simulink model "AirRefueling_Platform_PBVS_origin"  (R2022b)
settings: Solver=ode4  StartTime=0.0  StopTime=70  FixedStep=0.02  RelTol=1e-5  AbsTol=1e-4  EnableMultiTasking=on
InitFcn:
  | F16_Init
values from neighbouring files (symbols this model uses):
  airSpeed = 393.720000000000    (= 393.72)    [F16_Init.m]    (also in Initialization.m)
  alpha0 = trimAlpha*180/pi    (= 6.62393794015)    [F16_Init.m]    (also in Initialization.m)
  altitude = 9843    [F16_Init.m]    (also in Initialization.m)
  b_ref = 30.0    (= 30)    [F16_Init.m]    (also in Initialization.m)
  C = [ 1,0,0,zeros(1,15) ... (first row only)    [F16_Init.m]    (also in Initialization.m = [1,0,0,zeros(1,15))
  C2m = [C(1,:) ... (first row only)    [F16_Init.m]    (also in Initialization.m)
  d_f_rc = [3.75;0;-0.86]    [F16_Init.m]
  d_pr_rc = [6.06;0.54;-0.86]    [F16_Init.m]
  DeltaP = [0,0,DeltaP_z(j)]    [PBVS_main.m]
  dLEF = 0    [F16_Init.m]    (also in Initialization.m)
  fi_flag = 1    [F16_Init.m]    (also in Initialization.m)
  Kc = [ ... (first row only)    [F16_Init.m]    (also in Initialization.m)
  Ki = zeros(4,3)    [F16_Init.m]    (also in Initialization.m)
  Kp = zeros(4,18)    [F16_Init.m]    (also in Initialization.m)
  mass = 636.94    [F16_Init.m]    (also in Initialization.m)
  p0_rc = [-14.35-6.06-6;-0.54-(2);5.12+0.86-(-2)]    [F16_Init.m]
  q = zeros(N,1)    [hose3D_n_air_Fv_correction.m]
  trim_ail = 0.00874607850103852    (= 0.00874607850104)    [F16_Init.m]    (also in Initialization.m)
  trim_control = [trim_thrust;trim_ele;trim_ail;trim_rud]    [F16_Init.m]    (also in Initialization.m)
  trim_ele = -2.97973164860638    (= -2.97973164861)    [F16_Init.m]    (also in Initialization.m)
  trim_rud = 0.0680302158182712    (= 0.0680302158183)    [F16_Init.m]    (also in Initialization.m)
  trim_state1 = [trim_state;0;0;0;0;0;0]    [F16_Init.m]    (also in Initialization.m)
  trim_thrust = 2279.08519954656    (= 2279.08519955)    [F16_Init.m]    (also in Initialization.m)
undefined symbols (not defined in the file or in its folder): F, gray, MIL, vt0
libraries: aerolibconvert2 x6, aerolibasang x4, aerolibwind2 x2, aerolibobsolete x2, visionmorphops x2, vrlib x1, simulink x1, aerolibatmos2 x1, aerolibadyn x1, aerolibanimutils x1
(part 2 of 2)

== matlab function AirRefueling_Platform_PBVS_origin/SimToVR ==
  data: t input; y output; PosPr1 input; PosTb1 input
function y = SimToVR(t,PosPr1,PosTb1)
%#codegen

%%函数名：SimToVR
%%用途  ：将软管锥套坐标输出转换为VR输入
%%输入  ：PosPr - 受油机椎管坐标， PlsTb - 软管坐标数据
%%输出  ：VrPos - 软管和受油机VR位置，VrAngle - 旋转角度输出
%%作者  ：戴训华
%%时间  ：2014/3/19

PosPr = PosPr1(1:3);
AttitudeRecei = [PosPr1(4);-PosPr1(6);PosPr1(5)-0.115609];

PosTb = PosTb1(1:60);

VrAngle = zeros(22*4,1);
VrPos = zeros(22*3,1);


for j = 1:21                        %前20为软管坐标数据，后1为软管平滑过渡处理
    if j == 1
        pX = [0, 0, 0]';            %软管起点
        pY = PosTb(3*j-2:3*j);      %软杆终点
    elseif j == 21                  %多加一段杆，做过渡
        pX = PosTb(3*j-5:3*j-3);
        pY = [PosTb(3*j-5)-0.7163*cos(8/180*pi),PosTb(3*j-4),PosTb(3*j-3)+0.7163*sin(8/180*pi)]';
    else
        pX = PosTb(3*j-5:3*j-3);
        pY = PosTb(3*j-2:3*j); 
    end
    
    pZ = (pX + pY)/2;               %中点坐标
    pZ = pZ * 8/3;                  %到VR中比例的缩放

    vAxis = [0,0,-1]';               %水平轴
    vTb = pY - pX;                  %杆的方向
    
    axis1 = null([vAxis';vTb']);%获取垂直向量
    vRot = axis1(:,1)';             %得到旋转轴
    
    if vRot(2) < 0
        vRot = -vRot;
    end
    
    VrAngle(4*j-3:4*j-1) = [vRot(1),vRot(3),vRot(2)]';
    VrAngle(4*j) = acos(vAxis'*vTb / sqrt(vAxis'*vAxis * vTb'*vTb));
    
    VrPos(3*j-2:3*j) = [pZ(1),-pZ(3),pZ(2)]';
end
%y = u;
VrAngle(85:88)=[AttitudeRecei(1);AttitudeRecei(2);AttitudeRecei(3);norm(AttitudeRecei)];
pZ = PosPr+[0.35 -0.1 -0.05]';
pZ = pZ * 8/3;
VrPos(3*22-2:3*22) = [pZ(1),-pZ(3),pZ(2)]';

VrPos(3*21-2) = VrPos(3*21-2)+0.8;
VrPos(3*21-1) = VrPos(3*21-1)+0.1;

if t<10
    if t>1
        VrPos(1:21*3) = VrPos(1:21*3)*(t-1)/9;
    else
        VrPos(1:21*3) = VrPos(1:21*3)*0;
    end
end

y = [VrAngle;VrPos];

== matlab function AirRefueling_Platform_PBVS_origin/Hose-Drogue System/Bow Wave Effect/Bow Wave Effect Function ==
  data: x input; Fx output; y input; z input; Fy output; Fz output
function [Fx,Fy,Fz] = F_rc2dr(x,y,z)

Cx1 = 91.6170;
Cx2 = 0.3220;
Cx3 = 3.8870;
Cx4 = 2.7359;
Cx5 = 2.4939;
Cx6 = 309.7709;
Cx7 = 0.3237;
Cx8 = 0.3851;
Cx9 = 1.1471;

Cy1 = 223.3210;
Cy2 = 0.2082;
Cy3 = 0.8102;
Cy4 = 0.6555;

Cz1 = 173.2021;
Cz2 = 0.2141;
Cz3 = 0.5697;
Cz4 = 0.7038;

if x > 5.6493
    Fx = 0;
elseif x > 3.0893
    Fx = Cx1*(1-Cx2*(x-Cx3)^2)*exp(-y^2/Cx4)*exp(z/Cx5);
else
    Fx = Cx1*(1-Cx2*(x-Cx3)^2)*exp(-y^2/Cx4)*exp(z/Cx5)...
       + Cx6*(1-Cx7*x)*exp(-y^2/Cx8)*exp(z/Cx9);
end

if x > 4.8031
    Fy = 0;
else
    Fy = Cy1*(1-Cy2*x)*(y*exp(-y^2/Cy3))*exp(z/Cy4);
end

if x > 4.6275
    Fz = 0;
else
    Fz = -Cz1*(1-Cz2*x)*exp(-y^2/Cz3)*exp(z/Cz4);
end

== matlab function AirRefueling_Platform_PBVS_origin/Hose-Drogue System/Total Turbulence   ==
  data: u1 input; u input; y output
function y = Dr_wnd2Frc(u1,u)
%#codegen

Ve=120;
rho = 0.98;
Q=0.5*rho*Ve^2;
S=0.38;
CD=0.81*0.8;

uu=u(1);
vv=u(2);
ww=u(3);

%beta = acos(sqrt(vv^2+ww^2)/abs(uu));
%theta = atan(ww/vv);

C_beta = 0.3979;

yx=rho*S*CD*Ve*uu;
yy=Q*S*C_beta*vv/Ve;
yz=Q*S*C_beta*ww/Ve;


y = [yx,yy,yz]';
y=u1+y;

== matlab function AirRefueling_Platform_PBVS_origin/Visual Servo Block/MATLAB Function ==
  data: u input; y output
function y = fcn(u)
%#codegen

 Ir=u(:,:,1)*2-u(:,:,2)*1-u(:,:,3)*1;

% Ir=u(:,:,1)*0.3-u(:,:,2)*0.59-u(:,:,3)*0.11

S=size(Ir);
Iin=zeros(S(1),S(2));
for i=1:S(1)
    for j=1:S(2)
       if Ir(i,j)<50
            Iin(i,j)=0;
        else
            Iin(i,j)=1;
        end
    end
end


y = Iin;

== matlab function AirRefueling_Platform_PBVS_origin/Tanker System/   ==
  data: u input; y output
function y = WindTurFromTank(u)
%#codegen

y = TankerVortexWindField(u);

== matlab function AirRefueling_Platform_PBVS_origin/Visual Servo Block/MATLAB Function1 ==
  settings: updateMethod=DISCRETE
  data: u1 input; yy output; u2 input; u3 input; yy1 output; yy2 output; t input; AA data_store_memory; yytest output
%function [yy,yy1,yy2,posNdepth] = fcn(u1,u2,u3,t)
function [yy,yy1,yy2,yytest] = fcn(u1,u2,u3,t)
%#codegen
L=u1; %过滤后图像
N=u2; %识别出的目标点个数
Ir=u3; %原灰度图像
t0=0.1;
global AA;
%S=zeros(N,2);
dX=zeros(10,1);
dY=zeros(10,1);
 for k=1:N    %对所有出现的标志点进行计算，获得每个标志点图像坐标系下横纵坐标的平均下标位置。
     [r,c]=find(L == k);
     dX(k)=mean(r);   %r行数，也就是y坐标
     dY(k)=mean(c);   %c列数，也就是x坐标
 end
% %plot(S(:,1),S(:,2),'+')
% % dx(:,1)=S(:,1)-mean(S(:,1));
% % dy(:,1)=S(:,2)-mean(S(:,2));
% 
% dX=S(:,1);
% dY=S(:,2);

m=[dX(1:N,1) dY(1:N,1) ones(size(dX(1:N,1)))]\-(dX(1:N,1).^2+dY(1:N,1).^2);
% m = [dX(1:N,1) dY(1:N,1) ones(size(dX(1:N,1)))]的逆* -(dX(1:N,1).^2+dY(1:N,1).^2)
cX=-0.5*m(1);%目标锥套的圆心图像坐标以及半径（以左上点为坐标系原点的像素坐标系下的坐标以及半径长度）
cY=-0.5*m(2);
cR=sqrt((m(1)^2+m(2)^2)/4-m(3));%半径
if N==3
   AA=[cX;cY;cR]; 
end

if N<3
   cX=AA(1);
   cY=AA(2);
   cR=AA(3);
end

%yy=N;
% 
%yy = [cX,cY,cR];
%yy=[yy,N];


[mm,nn]=size(Ir);%图像视野大小  mm代表像素行数，nn代表像素列数。
%因为这里图像坐标系下横轴是x，纵轴是y。因此这里nn就是图像坐标系x轴坐标，mm就是图像坐标系y轴坐标。


if t>t0
    alpha=0:pi/100:2*pi;
    x=cR*cos(alpha)+cX;
    y=cR*sin(alpha)+cY;

    % if isempty(Ir)
    %     Ir=zeros(720,1280);    
    % end





    for k=1:length(alpha)

        i=floor(x(k));%取整
        j=floor(y(k));
        if(i>=1&&j>=1&&i<=mm&&j<=nn)
            Ir(i:i,j:j)=1;        
        end

    end
end    
    
if t>t0+0.05
    i=floor(cX);
    j=floor(cY);

    if(i-3>=1&&j-3>=1&&i+4<=mm&&j+4<=nn)
        Ir(i-3:i+4,j:j+1)=1; 
        Ir(i:i+1,j-3:j+4)=1;  
    end
end

if t>t0+0.1
    i=floor(mm/2+42.57);
    j=floor(44.14+nn/2);
    if(i-3>=1&&j-3>=1&&i+4<=mm&&j+4<=nn)
        Ir(i-3:i+4,j:j+1)=1; 
        Ir(i:i+1,j-3:j+4)=1;  
    end
end

yy=Ir;
% 
% 
% 
% 

yy1=[cY-nn/2,mm/2-cX,cR]; 
%yy1 以图像中心为原点的图像坐标系下的X,Y位置以及图像中半径长度。 这些均为像素长度，也就是矩阵里的下标个数。
%因为这里图像坐标系的y轴是向下的，因此这里yy1的y坐标就是mm/2-cX而不是cX-mm/2


%从像素坐标系转化为相机坐标系，相机坐标系下，x轴指向机头，y轴是图像坐标系下的x轴，z轴是图像坐标系下的y轴，因此这里有
%xw<-cR(yy1(2)), yw<-x(yy1(0)), zw<-y(yy1(1)).

f=196.8372/0.330;
s=196.8372/yy1(3);
xw=-s+1.928; %锥套的深度信息
yw=yy1(1)*s/f-(46.94*1.862225/f);
zw=yy1(2)*s/f+(52.06*1.862225/f)-0.02;



%ftest=196.8372/0.330;
xtest=s-1.928; %实际仿真最后对接成功，深度就是大约2.3.
ytest=yy1(1)*s/f-(46.94*1.862225/f);
ztest=-(yy1(2)*s/f+(52.06*1.862225/f));
yytest=[xtest,ytest,ztest];

yyw=-yw;
xxw=xw*cos(5/180*pi)-zw*sin(5/180*pi);
zzw=xw*sin(5/180*pi)-zw*cos(5/180*pi);

% xw=-s+1.8925;
% 
% yw=(yy1(1)*s/2/196.9344-0.2206)/-1.4705;
% zw=(yy1(2)*s/2/196.9344+0.4953-2.9364-1.4682*xw)/1.4682;
yy2=[xxw;yyw;zzw];
posNdepth=[xw;yw;zw];
% yy2=[xw;yw;zw];


% function [yy,yy1,yy2] = fcn(u1,u2,u3)
% %#codegen
% L=u1;
% N=u2;
% Ir=u3;
% %S=zeros(N,2);
% dX=zeros(10,1);
% dY=zeros(10,1);
%  for k=1:N
%      [r,c]=find(L == k);
%      dX(k)=mean(r);
%      dY(k)=mean(c);     
%  end
% % %plot(S(:,1),S(:,2),'+')
% % % dx(:,1)=S(:,1)-mean(S(:,1));
% % % dy(:,1)=S(:,2)-mean(S(:,2));
% % 
% % dX=S(:,1);
% % dY=S(:,2);
% 
% m=[dX(1:N,1) dY(1:N,1) ones(size(dX(1:N,1)))]\-(dX(1:N,1).^2+dY(1:N,1).^2);
% cX=-0.5*m(1);
% cY=-0.5*m(2);
% cR=sqrt((m(1)^2+m(2)^2)/4-m(3));
% 
% 
% %yy=N;
% % 
% %yy = [cX,cY,cR];
% %yy=[yy,N];
% 
% % 
% alpha=0:pi/100:2*pi;
% x=cR*cos(alpha)+cX;
% y=cR*sin(alpha)+cY;
% 
% % if isempty(Ir)
% %     Ir=zeros(720,1280);    
% % end
% 
% [mm,nn]=size(Ir);
% for k=1:length(alpha)
% 
%     i=floor(x(k));
%     j=floor(y(k));
%     if(i>=1&&j>=1&&i<=mm&&j<=nn)
%         Ir(i:i,j:j)=1;        
%     end
%         
% end
% 
% i=floor(cX);
% j=floor(cY);
% 
% if(i-3>=1&&j-3>=1&&i+4<=mm&&j+4<=nn)
%     Ir(i-3:i+4,j:j+1)=1; 
%     Ir(i:i+1,j-3:j+4)=1;  
% end
% 
% % 
% % 
% % 
% % 
% yy=Ir;
% 
% yy1=[cY-nn/2,mm/2-cX,cR];
% 
% s=196.9344/yy1(3);
% xw=-s+1.8925;
% 
% yw=(yy1(1)*s/2/196.9344-0.2206)/-1.4705;
% zw=(yy1(2)*s/2/196.9344+0.4953-2.9364-1.4682*xw)/1.4682;
% yy2=[xw;yw;zw];
% 
%

== matlab function AirRefueling_Platform_PBVS_origin/Visual Servo Block/MATLAB Function2 ==
  data: u input; y output
function y = fcn(u)
%#codegen

Ir=u(:,:,2)*2-u(:,:,1)*1-u(:,:,3)*1;

S=size(Ir);
Iin=zeros(S(1),S(2));
for i=1:S(1)
    for j=1:S(2)
       if Ir(i,j)<50
            Iin(i,j)=0;
        else
            Iin(i,j)=1;
       end
        
       if i/S(1)>0.8
           Iin(i,j)=0;
       end
       
    end
end


y = Iin;
